simulink model "sim_object_analysis"  (R2019a)
settings: Solver=ode23  StartTime=0.0  StopTime=400  RelTol=1e-3  EnableMultiTasking=on
values from neighbouring files (symbols this model uses):
  d = 0.5    [mod1s.m]
  h = 4    [mod1s.m]
  K = 19    [mod1s.m]
  T = 29    [mod1s.m]
settings Model: Creator=user  LastModifiedBy=ogure
settings SolverCC: InitialStep=10^-1  SolverResetMethod=Robust
settings DataIOCC: SaveFormat=Array  ReturnWorkspaceOutputs=off
settings OptimizationCC: LifeSpan=inf
settings DebuggingCC: SolverPrmCheckMsg=warning  SFUnexpectedBacktrackingDiag=warning  SFNoUnconditionalDefaultTransitionDiag=warning  SFExecutionAtInitializationDiag=none  ArithmeticOperatorsInVariantConditions=warning
settings HardwareCC: ProdBitPerPointer=32  ProdBitPerSizeT=32  ProdBitPerPtrDiffT=32  ProdLargestAtomicFloat=None  ProdIntDivRoundTo=Undefined  ProdEndianess=Unspecified  ProdWordSize=32  ProdHWDeviceType=32-bit Generic
settings ModelReferenceCC: PropagateSignalLabelsOutOfModel=off
settings SFSimCC: SimUseLocalCustomCode=off
settings RTWCC: RTWUseLocalCustomCode=off
settings CodeAppCC: StateflowObjectComments=on
settings GRTTargetCC: TargetLangStandard=C89/C90 (ANSI)  GeneratePreprocessorConditionals=Disable all
settings ConfigComp: CovMetricSettings=dw  CovHtmlReporting=on  CovSaveCumulativeToWorkspaceVar=on  CovSaveSingleToWorkspaceVar=on  CovExternalEMLEnable=off  CovSFcnEnable=off

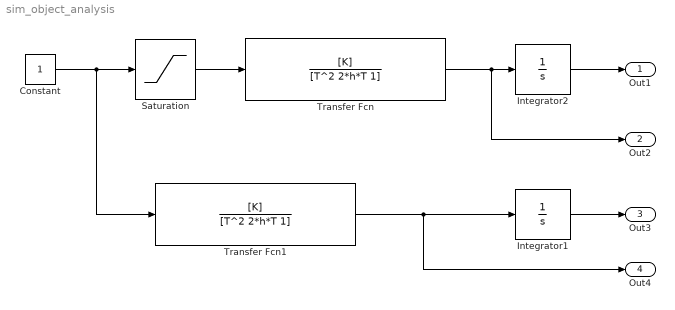
== system sim_object_analysis ==
  Constant : Constant
  Integrator1 : Integrator
  Integrator2 : Integrator
  Saturation : Saturate  UpperLimit=d  LowerLimit=-d
  Transfer Fcn : TransferFcn  Numerator=[K]  Denominator=[T^2 2*h*T 1]
  Transfer Fcn1 : TransferFcn  Numerator=[K]  Denominator=[T^2 2*h*T 1]
  Out1 : Outport  SignalName=x
  Out2 : Outport  Port=2  SignalName=y
  Out3 : Outport  Port=3  SignalName=x1
  Out4 : Outport  Port=4  SignalName=y1
  wires:
  Constant/1 -> Transfer Fcn1/1, Saturation/1
  Transfer Fcn1/1 -> Out4/1, Integrator1/1
  Transfer Fcn/1 -> Out2/1, Integrator2/1
  Integrator2/1 -> Out1/1
  Saturation/1 -> Transfer Fcn/1
  Integrator1/1 -> Out3/1
